simulink model "shiftcontrol72mod2"  (R2021a)
settings: Solver=VariableStepAuto  StartTime=0.0  StopTime=10.0  RelTol=1e-3
libraries: spsMultimeterLib x2, spsDCVoltageSourceLib x1, spsGroundLib x1, spsPWMGenerator2LevelLib x1, spsSeriesRLCBranchLib x1, dspsrcs4 x1, spsUniversalBridgeLib x1, spspowerguiLib x1
settings Model: Creator=User  LastModifiedBy=User

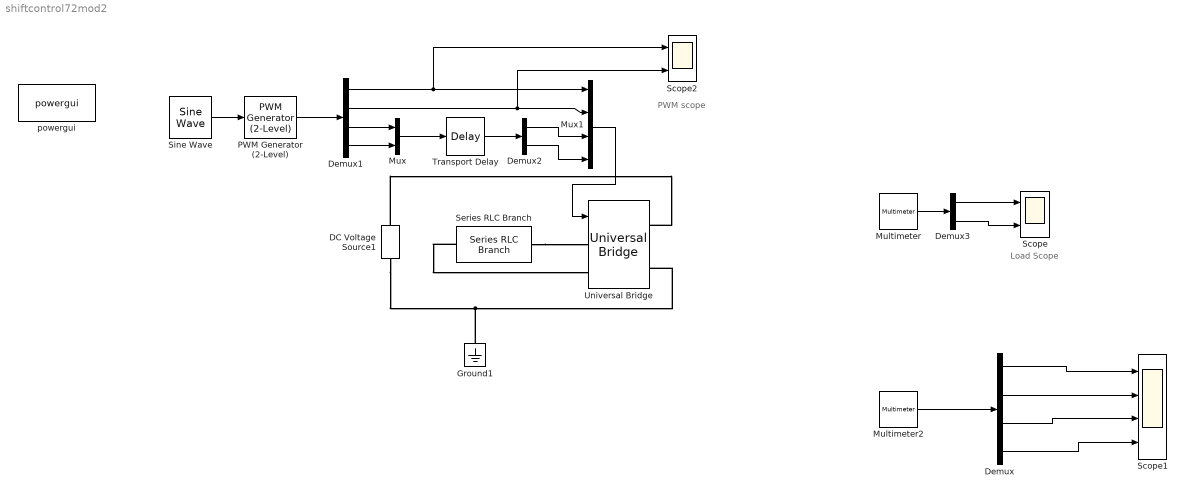
== system shiftcontrol72mod2 ==
  note: PWM scope
  note: Load Scope
  DC Voltage Source1 : spsDCVoltageSourceLib/DC Voltage Source  Amplitude=200  Measurements=None
  Demux : Demux
  Demux1 : Demux
  Demux2 : Demux  Outputs=2
  Demux3 : Demux  Outputs=2
  Ground1 : spsGroundLib/Ground  LConnTagsString=a
  Multimeter : spsMultimeterLib/Multimeter  PhasorSimulation=off  OutputType=Complex  sel=[1 8]  L=12  Gain=[1 1]  yselected={'Ub: Series RLC Branch','Ib: Series RLC Branch'};  PSBOutputType=1  PSBequivalent=0  AxesSetting=[0,0.1,-100,100]  Display=0  SavedBlockNames=-11
  Multimeter2 : spsMultimeterLib/Multimeter  PhasorSimulation=off  OutputType=Complex  sel=[2 3 9 10]  L=12  Gain=[1 1 1 1]  yselected={'Usw1: Universal Bridge','Usw2: Universal Bridge','Isw1: Universal Bridge','Isw2: Universal Bridge'};  PSBOutputType=1  PSBequivalent=0  AxesSetting=[0,0.1,-100,100]  Display=0  SavedBlockNames=-11
  Mux : Mux  Inputs=2
  Mux1 : Mux
  PWM Generator (2-Level) : spsPWMGenerator2LevelLib/PWM Generator (2-Level)  ModulatorType=Single-phase full-bridge (4 pulses)  ModulatorMode=Unsynchronized  Fc=50  Pc=-90  nF=27  MinMax="[ -1  1 ]"  SamplingTechnique=Natural  ModulatingSignals=off  m=0.8  Freq=60  Phase=0  Ts=0  ShowCarrierOutport=off
  Scope : Scope  NumInputPorts=2
  Scope1 : Scope  NumInputPorts=4
  Scope2 : Scope  NumInputPorts=2
  Series RLC Branch : spsSeriesRLCBranchLib/Series RLC Branch  LConnTagsString=__new0  RConnTagsString=__new0  BranchType=RL  Resistance=100  Inductance=1  SetiL0=off  InitialCurrent=0  Capacitance=1e-6  Setx0=off  InitialVoltage=0  Measurements=Branch voltage and current
  Sine Wave : dspsrcs4/Sine Wave  Amplitude=2  Frequency=50  Phase=0  SampleMode=Discrete  OutComplex=Real  CompMethod=Trigonometric fcn  TableSize=Speed  SampleTime=1/1000  SamplesPerFrame=1  ResetState=Restart at time zero  OutputFrames=off  dataType=double  wordLen=16  udDataType=sfix(16)  fracBitsMode=Best precision  numFracBits=15  OutDataTypeStr=double  LastOutDataTypeStr=double
  Transport Delay : TransportDelay  DelayTime=72*0.01/180
  Universal Bridge : spsUniversalBridgeLib/Universal Bridge  Arms=2  SnubberResistance=1e5  SnubberCapacitance=inf  Device=IGBT / Diodes  Ron=1e-3  Lon=0  ForwardVoltages="[  0  0  ]"  ForwardVoltage=0  GTOparameters=[ 10e-6 , 20e-6 ]  IGBTparameters=[ 1e-6 , 2e-6 ]  Measurements=All voltages and currents  Measurements_2=None  converterType=Rectifier
  powergui : spspowerguiLib/powergui  Priority=1  SimulationMode=Discrete  SampleTime=5e-5  frequency=60  Iterations=50  frequencyindice=0  Pbase=100e6  ErrMax=1e-4  UnitsV=kV  UnitsW=MW  buscounter=0  FunctionMessages=off  echomessages=off  EnableUseOfTLC=off  CurrentSourceSwitches=off  DisableSnubberDevices=off  DisableRonSwitches=off  DisableVfSwitches=off  DisplayEquations=off  AutomaticDiscreteSolvers=off  SolverType=Tustin/Backward Euler (TBE)  Interpol=off  ExternalGateDelay=off  methode=off  Ts=100  x0status=blocks  SPID=on  SwTol=0  HookPort=off  NonlinearTolerance=1e-4  nMaxIteration=100  ContinueOnMaxIteration=off  RestoreLinks=warning  ResistiveCurrentMeasurement=off  Frange=[0:2:500]  Ylog=off  Xlog=on  ShowGrid=off  save=off  variable=ZData  structure=0  ZoomFFT=off  StartTime=0.0  cycles=1  DisplayStyle=1  fundamental=60  FreqAxis=off  MaxFrequency=1000  frequencyindicesteady=1  RmsSteady=1  display=off
  wires:
  Demux/3 -> Scope1/3
  Demux/1 -> Scope1/1
  Demux/2 -> Scope1/2
  Multimeter2/1 -> Demux/1
  Demux/4 -> Scope1/4
  Sine Wave/1 -> PWM Generator (2-Level)/1
  PWM Generator (2-Level)/1 -> Demux1/1
  Demux1/3 -> Mux/1
  Demux1/4 -> Mux/2
  Mux/1 -> Transport Delay/1
  Transport Delay/1 -> Demux2/1
  Demux1/1 -> Scope2/1, Mux1/1
  Demux1/2 -> Scope2/2, Mux1/2
  Demux2/1 -> Mux1/3
  Demux2/2 -> Mux1/4
  Mux1/1 -> Universal Bridge/1
  Multimeter/1 -> Demux3/1
  Demux3/1 -> Scope/1
  Demux3/2 -> Scope/2
  connections:
  DC Voltage Source1/RConn1 -- Universal Bridge/RConn1
  DC Voltage Source1/LConn1 -- Ground1/LConn1 -- Universal Bridge/RConn2
  Series RLC Branch/RConn1 -- Universal Bridge/LConn1
  Series RLC Branch/LConn1 -- Universal Bridge/LConn2
